simulink model "tutorial3"  (Simulink 2.20)
settings: Solver=ode5  StartTime=0.0  StopTime=tstop  FixedStep=tstep  MaxStep=tstep  RelTol=1e-3  AbsTol=1e-3
values from neighbouring files (symbols this model uses):
  a = a    [buttfilt.m]
settings Model: SaveTime=off  SaveOutput=off  ConsistencyChecking=off  RTWPlaceOutputsASAP=off

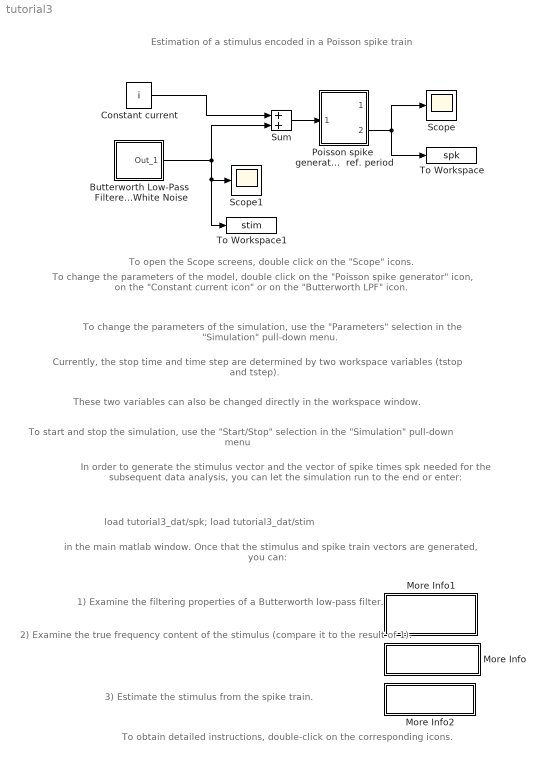
== system tutorial3 ==
  note: Estimation of a stimulus encoded in a Poisson spike train
  note: To change the parameters of the model, double click on the
      | "Poisson spike generator" icon, on the "Constant current icon"
      | or on the "Butterworth LPF" icon.
  note: To open the Scope screens, double click on the "Scope" icons.
  note: To change the parameters of the simulation, use the "Parameters"
      | selection in the "Simulation" pull-down menu.
  note: Currently, the stop time and time step are determined by two
      | workspace variables (tstop and tstep).
  note: These two variables can also be changed directly in the
      | workspace window.
  note: To start and stop the simulation, use the "Start/Stop"
      | selection in the "Simulation" pull-down menu
  note: In order to generate the stimulus vector and the vector of spike times
      | spk needed for the subsequent data analysis, you can let the simulation
      | run to the end or enter:
  note: load tutorial3_dat/spk; load tutorial3_dat/stim
  note: in the main matlab window. Once that the stimulus and spike train
      | vectors are generated, you can:
  note: 1) Examine the filtering properties of a Butterworth
      | low-pass filter.
  note: 2) Examine the true frequency content of the
      | stimulus (compare it to the result of 1).
  note: 3) Estimate the stimulus from the spike train.
  note: To obtain detailed instructions, double-click on the corresponding
      | icons.
  Butterworth Low-Pass  Filtered White Noise : Subsystem  mask(Low-pass filtered white noise. ){@1=tstep, @2=0.6, @3=[23341], @4=40, @5=4}
      mask prompts: @1 "time step [msec]"; @2 "standard deviation [nA]"; @3 "random seed"; @4 "Cut-off frequency [Hz]"; @5 "filter order"
      mask help: Discrete time white noise
      mask init:
      | dt = @1; sigma = @2; seed = @3;[bint, a] = butter(@5,@4*2*@1*1e-3); h = freqz(bint,a); nfac = sum(h.*conj(h))/length(h); b = bint/sqrt(nfac); n = @5; x = rand(1,10*@5); y = filter(b,a,x);
      mask Help: Generates a Gaussian noise with fixed standard deviation  in the time domain and fixed cut-off frequency in the frequency domain.
      mask Display: plot((5*n:10*n),y(5*n:10*n));
  Constant current : Constant  Value=i  mask(constant current){@1=0.6}
      mask prompts: @1 "constant current value [nA]"
      mask help: Parameter
      mask init:
      | i = @1;
      mask Help: Provides a constant input current
  More Info : Subsystem
      mask Display: disp('Stimulus power\nspectrum')
  More Info1 : Subsystem
      mask Display: disp('Butterworth\nlow-pass filter\nproperties')
  More Info2 : Subsystem
      mask Display: disp('Stimulus\nestimation')
  Poisson spike  generator with  ref. period : Subsystem  mask(I&F p. thres., ref. per.){@1=tstep, @2=10, @3=.5, @4=5}
      mask prompts: @1 "time step [msec]"; @2 "mean threshold [mV]"; @3 "Capacitance [nF]"; @4 "refractory period [msec]"
      mask help: Parameters
      mask init:
      | dt = @1; thres = @2; C = @3; ref = @4;
      mask Help: For a detailled description of the model, please type 'help piandfr' in the main matlab window
      mask Display: disp('Vm \n\n spikes')
  Scope : Scope
      settings: TickLabels=on  TimeRange=500.000000  YMin=-2.000000  YMax=2.000000  SaveToWorkspace=off  SaveName=ScopeData
  Scope1 : Scope
      settings: TickLabels=on  TimeRange=500.000000  YMin=-2.000000  YMax=2.000000  SaveToWorkspace=off  SaveName=ScopeData
  Sum : Sum  Inputs=++
  To Workspace : ToWorkspace  VariableName=spk  SampleTime=0
      settings: Buffer=ceil(tstop/tstep)
  To Workspace1 : ToWorkspace  VariableName=stim  SampleTime=0
      settings: Buffer=ceil(tstop/tstep)
  wires:
  Sum/1 -> Poisson spike  generator with  ref. period/1(in_1)
  Poisson spike  generator with  ref. period/2(out_1) -> To Workspace/1, Scope/1
  Constant current/1 -> Sum/1
  Butterworth Low-Pass  Filtered White Noise/1(Out_1) -> Sum/2, Scope1/1, To Workspace1/1

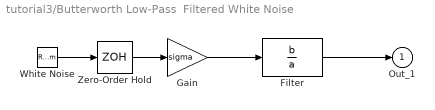
== system tutorial3/Butterworth Low-Pass  Filtered White Noise ==
  Filter : DiscreteFilter  Numerator=b  Denominator=a  SampleTime=dt
  Gain : Gain  Gain=sigma
  White Noise : RandomNumber  Mean=0  Variance=1  Seed=seed  SampleTime=-1
  Zero-Order Hold : ZeroOrderHold  SampleTime=dt
  Out_1 : Outport  Port=1  InitialOutput=0
  wires:
  Zero-Order Hold/1 -> Gain/1
  White Noise/1 -> Zero-Order Hold/1
  Filter/1 -> Out_1/1
  Gain/1 -> Filter/1

== system tutorial3/More Info ==
  note: To compute the power spectrum and
      | autocorrelation of the stimulus, enter:
  note: psautostim(stim,tstep)
  note: in the workspace window.

== system tutorial3/More Info1 ==
  note: To see the transfer characteristics of a Butterworth
      | low pass filter, enter:
  note: buttfilt(40,4,tstep)
  note: The parameters are:
  note: 40 = cut-off frequency of the filter
  note: 4 = order of the filter
  note: tstep = time step for the simulation
  note: in the workspace window.

== system tutorial3/More Info2 ==
  note: To obtain an estimate of the stimulus from the spike
      | train and to quantify the reliability of the encoding, enter
  note: stimest(stim,spk,tstep)
  note: in the workspace window.

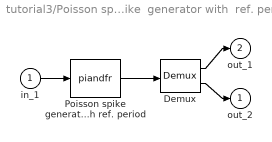
== system tutorial3/Poisson spike  generator with  ref. period ==
  in_1 : Inport  Port=1  PortWidth=-1  SampleTime=-1
  Demux : Demux  Outputs=2
  Poisson spike generator with ref. period : S-Function  FunctionName=piandfr  Parameters=dt,thres,C, ref  PortCounts=[]  SFunctionModules=''
  out_2 : Outport  Port=1  InitialOutput=0
  out_1 : Outport  Port=2  InitialOutput=0
  wires:
  Poisson spike generator with ref. period/1 -> Demux/1
  Demux/1 -> out_1/1
  Demux/2 -> out_2/1
  in_1/1 -> Poisson spike generator with ref. period/1
